simulink model "SPWM"  (R2023a)
settings: Solver=VariableStepAuto  StartTime=0.0  StopTime=0.5  RelTol=1e-3
libraries: spsMosfetLib x4, spsVoltageMeasurementLib x2, spsDCVoltageSourceLib x1, spspowerguiLib x1, spsSeriesRLCBranchLib x1, spsTHDLib x1, spsTriangleGeneratorLib x1
settings Model: Creator=vande  LastModifiedBy=vande
settings DataIOCC: ReturnWorkspaceOutputs=off

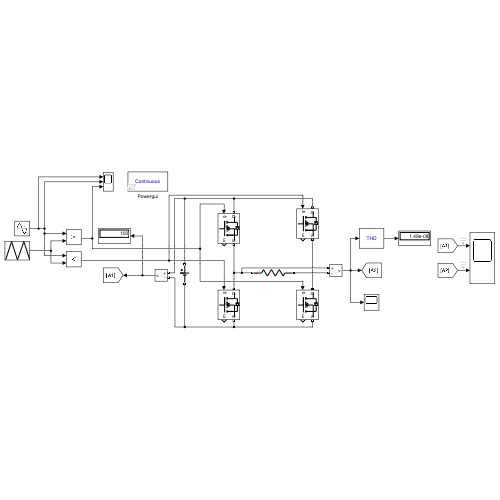
[thumbnail: Simulink's stored preview of the top-level diagram]
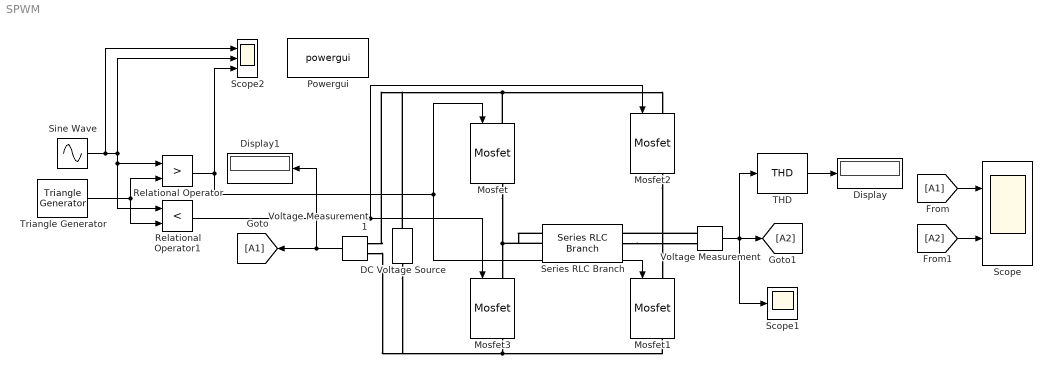
== system SPWM ==
  DC Voltage Source : spsDCVoltageSourceLib/DC Voltage Source  Amplitude=100  Measurements=None
  Display : Display
  Display1 : Display
  Mosfet{,1..3} (4 alike) : spsMosfetLib/Mosfet  Ron=0.1  Lon=0  Rd=0.01  Vfd=0  IC=0  Rs=1e5  Cs=inf  Measurements=on
  Powergui : spspowerguiLib/powergui  Priority=1  SimulationMode=Continuous  SampleTime=50e-6  frequency=60  Iterations=50  frequencyindice=0  Pbase=100e6  ErrMax=1e-4  UnitsV=kV  UnitsW=MW  buscounter=0  FunctionMessages=off  echomessages=off  EnableUseOfTLC=off  CurrentSourceSwitches=off  DisableSnubberDevices=off  DisableRonSwitches=off  DisableVfSwitches=off  DisplayEquations=off  AutomaticDiscreteSolvers=off  SolverType=Tustin/Backward Euler (TBE)  Interpol=off  ExternalGateDelay=off  methode=off  Ts=100  x0status=blocks  SPID=on  SwTol=0  HookPort=off  NonlinearTolerance=1e-4  nMaxIteration=100  ContinueOnMaxIteration=off  RestoreLinks=warning  ResistiveCurrentMeasurement=off  Frange=[0:2:500]  Ylog=off  Xlog=on  ShowGrid=off  save=off  variable=ZData  structure=0  ZoomFFT=off  StartTime=0.0  cycles=1  DisplayStyle=1  fundamental=60  FreqAxis=off  MaxFrequency=1000  frequencyindicesteady=1  RmsSteady=1  display=off
  Relational Operator : RelationalOperator  Operator=>  OutDataTypeStr=boolean  RndMeth=Simplest  InputSameDT=off
  Relational Operator1 : RelationalOperator  Operator=<  OutDataTypeStr=boolean  RndMeth=Simplest  InputSameDT=off
  Scope : Scope  NumInputPorts=2
  Scope1 : Scope
  Scope2 : Scope  NumInputPorts=3
  Series RLC Branch : spsSeriesRLCBranchLib/Series RLC Branch  LConnTagsString=__new0  RConnTagsString=__new0  BranchType=R  Resistance=30  Inductance=1e-3  SetiL0=off  InitialCurrent=0  Capacitance=1e-6  Setx0=off  InitialVoltage=0  Measurements=None
  Sine Wave : Sin  Amplitude=10  Frequency=314  SampleTime=0
  THD : spsTHDLib/THD  Freq=60  Ts=0
  Triangle Generator : spsTriangleGeneratorLib/Triangle Generator  Freq=100  Phase=0  Ts=0
  Voltage Measurement : spsVoltageMeasurementLib/Voltage Measurement  PhasorSimulation=off  OutputType=Complex  PSBequivalent=0
  Voltage Measurement1 : spsVoltageMeasurementLib/Voltage Measurement  PhasorSimulation=off  OutputType=Complex  PSBequivalent=0
  wires:
  Voltage Measurement/1 -> [A2], Scope1/1, THD/1
  [A2] -> Scope/2
  Voltage Measurement1/1 -> [A1], Display1/1
  THD/1 -> Display/1
  [A1] -> Scope/1
  Sine Wave/1 -> Scope2/1, Relational Operator1/1, Relational Operator/1, Scope2/2
  Triangle Generator/1 -> Relational Operator/2, Relational Operator1/2
  Relational Operator/1 -> Mosfet1/1, Mosfet/1, Scope2/3
  Relational Operator1/1 -> Mosfet3/1, Mosfet2/1
  connections:
  Series RLC Branch/RConn1 -- Voltage Measurement/LConn2
  Mosfet/LConn1 -- DC Voltage Source/RConn1 -- Voltage Measurement1/LConn1 -- Mosfet2/LConn1
  Mosfet3/RConn1 -- DC Voltage Source/LConn1 -- Voltage Measurement1/LConn2 -- Mosfet1/RConn1
  Mosfet/RConn1 -- Mosfet3/LConn1 -- Series RLC Branch/LConn1 -- Voltage Measurement/LConn1
  Mosfet2/RConn1 -- Mosfet1/LConn1
